simulink model "axis_video_signal_gen"  (R2025a)
settings: Solver=VariableStepAuto  StartTime=0.0  StopTime=gen_duration  RelTol=1e-3
PreLoadFcn:
  | AXI_video_stream_sig_gen_setup
InitFcn:
  | AXI_video_stream_sig_gen_setup
StartFcn:
  | AXI_video_stream_sig_gen_setup
StopFcn:
  | signal_set = out;
  | 
  | save('AXI_video_stream_sig.mat', '-v7.3', 'signal_set')
values from neighbouring files (symbols this model uses):
  fs = 100e6    (= 100000000)    [setup.m]
libraries: visionhdlio x1, visionsources x1
settings Model: Creator=fsb21125  LastModifiedBy=fsb21125

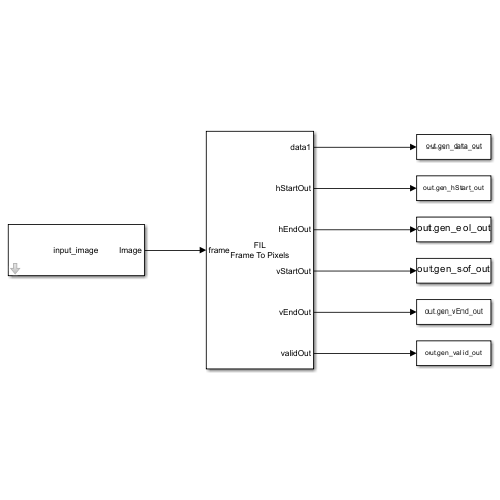
[thumbnail: Simulink's stored preview of the top-level diagram]
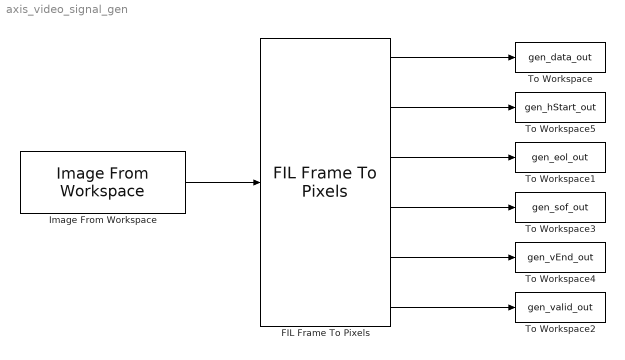
== system axis_video_signal_gen ==
  FIL Frame To Pixels : visionhdlio/FIL Frame To Pixels  NumComponents=1  NumPixels=8  OutputVectorFormat=Pixel  VideoFormat=Custom  ActivePixelsPerLine=320  ActiveVideoLines=240  TotalPixelsPerLine=408  TotalVideoLines=328  StartingActiveLine=1  FrontPorch=48  SampleTime=0  VideoFormatCache=Custom  ActivePixelsPerLineCache=320  ActiveVideoLinesCache=240  TotalPixelsPerLineCache=408  TotalVideoLinesCache=328  StartingActiveLineCache=1  FrontPorchCache=48
  Image From Workspace : visionsources/Image From Workspace  Tag=vipblks_nd  ImageValue=input_image  Ts=1/fs  imagePorts=One multidimensional signal  OutPortLabels=R|G|B  ImageDataType=Inherit from 'Value'  Signed=on  WordLength=16  sdImageDataType=sfix(16)  FractionLengthMode=User-defined  FractionLength=15
  To Workspace : ToWorkspace  VariableName=gen_data_out  SampleTime=-1
      settings: Save2DSignal=2-D array (concatenate along first dimension)
  To Workspace1 : ToWorkspace  VariableName=gen_eol_out  SampleTime=-1
      settings: Save2DSignal=2-D array (concatenate along first dimension)
  To Workspace2 : ToWorkspace  VariableName=gen_valid_out  SampleTime=-1
      settings: Save2DSignal=2-D array (concatenate along first dimension)
  To Workspace3 : ToWorkspace  VariableName=gen_sof_out  SampleTime=-1
      settings: Save2DSignal=2-D array (concatenate along first dimension)
  To Workspace4 : ToWorkspace  VariableName=gen_vEnd_out  SampleTime=-1
      settings: Save2DSignal=2-D array (concatenate along first dimension)
  To Workspace5 : ToWorkspace  VariableName=gen_hStart_out  SampleTime=-1
      settings: Save2DSignal=2-D array (concatenate along first dimension)
  wires:
  Image From Workspace/1 -> FIL Frame To Pixels/1
  FIL Frame To Pixels/1 -> To Workspace/1
  FIL Frame To Pixels/6 -> To Workspace2/1
  FIL Frame To Pixels/4 -> To Workspace3/1
  FIL Frame To Pixels/3 -> To Workspace1/1
  FIL Frame To Pixels/5 -> To Workspace4/1
  FIL Frame To Pixels/2 -> To Workspace5/1
